simulink model "Citation_FlightGear"  (R2020b)
settings: Solver=ode5  StartTime=0.0  StopTime=100  FixedStep=0.01  RelTol=1e-3  EnableMultiTasking=on
values from neighbouring files (symbols this model uses):
  cv1 = 20000    [gear_params.m]
  cv2 = cv1    (= 20000)    [gear_params.m]
  cv3 = 4000    [gear_params.m]
  cv4 = 20000    [gear_params.m]
  deltagmax1 = 0.25    [gear_params.m]
  deltagmax2 = deltagmax1    (= 0.25)    [gear_params.m]
  deltagmax3 = 0.24    [gear_params.m]
  deltagmax4 = 0.02    [gear_params.m]
  kt1 = 525020    [gear_params.m]
  kt2 = kt1    (= 525020)    [gear_params.m]
  kt3 = 457050    [gear_params.m]
  murol = 0.03*10    (= 0.3)    [gear_params.m]
  P1 = 2000    [gear_params.m]
  P2 = P1    (= 2000)    [gear_params.m]
  P3 = 2550    [gear_params.m]
  P4 = 40000    [gear_params.m]
  xl1 = xcg-6.858    [gear_params.m]
  xl2 = xcg-6.858    [gear_params.m]
  xl3 = xcg-2.0752    [gear_params.m]
  xl4 = xcg-12.742    [gear_params.m]
  yl1 = 1.918    [gear_params.m]
  yl2 = -1.918    [gear_params.m]
  yl3 = 0    [gear_params.m]
  yl4 = 0    [gear_params.m]
  zl1 = zcg-1.701    [gear_params.m]
  zl2 = zcg-1.701    [gear_params.m]
  zl3 = zcg-1.7488    [gear_params.m]
  zl4 = zcg-2.78    [gear_params.m]
undefined symbols (not defined in the file or in its folder): chord, Deng, ealphag, ealphas, Earth, g0, hDME, hGS, lh, massinit, matbuaf, matdaf, matdam, matdbbf, matdeaf, matdgaf, matdqaf, matduaf, matdwaw, matedhr, mateif, matelhr, matemhr, matemv1, matemv2, matemve, matetam, mateuaf, matfaaf, matfaxl, matff, matibaf, matibb, matibmh, matipaf, matipmh, matiraf, matiuaf, matiwaf, matlaf, matlam, matleaf, matleam, matlgaf, matlqaf, matluaf, matmaaf, matmaam, matmaf, matmam, matmbbf, matmeaf, matmeam, matmgaf, matmqaf, matmrbr, matn1d, matn2d, matnbab, matnbaf ... (+55)
libraries: aerolibfltsims x3, aerolibconvert2 x2, aerolibtransform2 x1, aerolibobsolete x1, vrlib x1, aerolibanimutils x1
(part 1 of 5)
settings Model: ExtModeTrigMode=oneshot  ExtModeArmWhenConnect=off  Creator=laurensvaneykeren  LastModifiedBy=ccdevisser
settings DataIOCC: SaveFormat=Array  SignalLoggingSaveFormat=ModelDataLogs  ReturnWorkspaceOutputs=off  SignalLoggingName=sigsOut
settings OptimizationCC: BooleanDataType=off  ExpressionDepthLimit=2147483647  LifeSpan=inf
settings DebuggingCC: SaveWithParameterizedLinksMsg=none  UnderspecifiedInitializationDetection=Classic  MergeDetectMultiDrivingBlocksExec=none  SignalResolutionControl=TryResolveAllWithWarning  MultiTaskDSMMsg=warning  MultiTaskCondExecSysMsg=none  FcnCallInpInsideContextMsg=warning  StateNameClashWarn=warning  SFUnexpectedBacktrackingDiag=warning  SFNoUnconditionalDefaultTransitionDiag=warning  SFExecutionAtInitializationDiag=none  ArithmeticOperatorsInVariantConditions=warning
settings HardwareCC: ProdBitPerPointer=32  ProdBitPerSizeT=32  ProdBitPerPtrDiffT=32  ProdLargestAtomicFloat=None  ProdIntDivRoundTo=Undefined  ProdEndianess=Unspecified  ProdWordSize=32  ProdHWDeviceType=32-bit Generic  TargetUnknown=on
settings ModelReferenceCC: PropagateSignalLabelsOutOfModel=off
settings SFSimCC: SimUseLocalCustomCode=off  CustomCodeUndefinedFunction=UseInterfaceOnly
settings RTWCC: SystemTargetFile=grt_malloc.tlc  GenCodeOnly=on  TemplateMakefile=grt_malloc_default_tmf  RTWUseLocalCustomCode=off
settings CodeAppCC: StateflowObjectComments=on
settings GRTTargetCC: TargetLangStandard=C89/C90 (ANSI)  CombineOutputUpdateFcns=off  GRTInterface=on  UseMalloc=on
settings ConfigComp: CovMetricSettings=dw  CovSaveCumulativeToWorkspaceVar=on  CovSaveSingleToWorkspaceVar=on

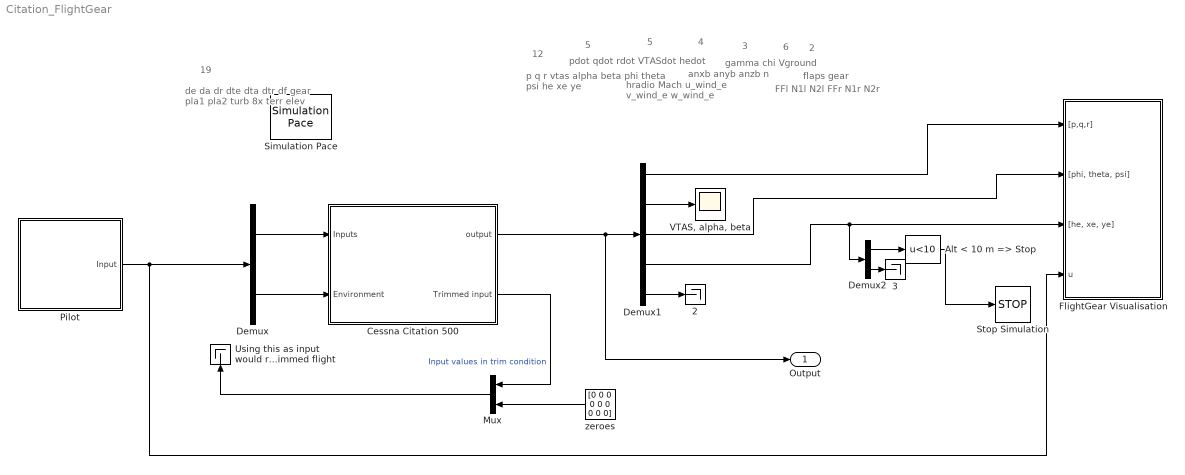
== system Citation_FlightGear ==
  note: de
      | da
      | dr
      | dte
      | dta
      | dtr
      | df
      | gear
      | pla1
      | pla2
      | turb 8x
      | terr elev
  note: p
      | q
      | r
      | vtas
      | alpha
      | beta
      | phi
      | theta
      | psi
      | he
      | xe
      | ye
  note: pdot
      | qdot
      | rdot
      | VTASdot
      | hedot
  note: hradio
      | Mach
      | u_wind_e
      | v_wind_e
      | w_wind_e
  note: anxb
      | anyb
      | anzb
      | n
  note: gamma
      | chi
      | Vground
  note: flaps
      | gear
  note: FFl
      | N1l
      | N2l
      | FFr
      | N1r
      | N2r
  note: 12
  note: 5
  note: 5
  note: 4
  note: 3
  note: 6
  note: 2
  note: 19
  2 : Terminator
  3 : Terminator
  Alt < 10 m => Stop : Fcn  Expr=u<10
  Cessna Citation 500 : Subsystem  mask(Citation Aircraft Model){trimdatafile=CitTrim_V140_H10500_M5300.tri}
      mask prompts: trimdatafile "Trim Condition"
      mask init:
      | initcit;
      mask Display:
      | image(imread('Citation.jpg'))
      | port_label('input', 1, 'Inputs')
      | port_label('input', 2, 'Environment')
      | port_label('output', 1, 'Outputs')
      | port_label('output', 2, 'Trim inputs')
  Demux : Demux  Outputs=[10 9]
      settings: DisplayOption=none
  Demux1 : Demux  Outputs=[3 3 3 3 25]
      settings: DisplayOption=none
  Demux2 : Demux  Outputs=[1 2]
  FlightGear Visualisation : Subsystem
  Mux : Mux  Inputs=2
  Pilot : Subsystem
  Simulation Pace : aerolibanimutils/Simulation Pace  SimulationPace=1  SleepMode=MATLAB Thread  OutputPaceError=off  SampleTime=-1
      settings: AttributesFormatString=%<SimulationPace> sec/sec
  Stop Simulation : Stop
  Using this as input would result in trimmed flight : Terminator
  "VTAS, alpha, beta" : Scope
  zeroes : Constant  Value=[0 0 0 0 0 0 0 0 0]
  Output : Outport
  wires:
  Demux/1 -> Cessna Citation 500/1(Inputs)
  Cessna Citation 500/1(output) -> Demux1/1, Output/1
  Demux/2 -> Cessna Citation 500/2(Environment)
  Cessna Citation 500/2(Trimmed input) -> Mux/1  "Input values in trim condition"
  zeroes/1 -> Mux/2
  Mux/1 -> Using this as input would result in trimmed flight/1
  Demux1/1 -> FlightGear Visualisation/1("[p,q,r]")
  Demux1/2 -> "VTAS, alpha, beta"/1
  Alt < 10 m => Stop/1 -> Stop Simulation/1
  Demux1/5 -> 2/1
  Demux1/4 -> Demux2/1, FlightGear Visualisation/3("[he, xe, ye]")
  Demux2/1 -> Alt < 10 m => Stop/1
  Pilot/1(Input) -> FlightGear Visualisation/4(u), Demux/1
  Demux2/2 -> 3/1
  Demux1/3 -> FlightGear Visualisation/2(" [phi, theta, psi]")

== system Citation_FlightGear/Cessna Citation 500 ==
  note: p
      | q
      | r
      | vtas
      | alpha
      | beta
      | phi
      | theta
      | psi
      | he
      | xe
      | ye
  note: de
      | da
      | dr
      | dte
      | dta
      | dtr
      | df
      | gear
      | pla1
      | pla2
  note: pdot
      | qdot
      | rdot
      | VTASdot
      | hedot
  note: hradio
      | Mach
      | u_wind_e
      | v_wind_e
      | w_wind_e
  note: anxb
      | anyb
      | anzb
      | n
  note: gamma
      | chi
      | Vground
  note: turb 8x
      | terr_elev
  note: flaps
      | gear
  note: de
      | da
      | dr
      | dte
      | dta
      | dtr
      | df
      | gear
      | pla1
      | pla2
  note: FFl
      | N1l
      | N2l
      | FFr
      | N1r
      | N2r
  Inputs : Inport
  Environment : Inport  Port=2
  Actuators : Subsystem
  Citation model DASMAT : Subsystem
  Controllers : Subsystem
  Demux4 : Demux  Outputs=[8 2]
      settings: DisplayOption=none
  Mux1 : Mux  Inputs=7
  Mux2 : Mux  Inputs=2
  trim conditions : Subsystem
  ua sel : Selector  IndexOptions=Index vector (dialog)  Indices=[5 6]  OutputSizes=1
  xdot sel : Selector  IndexOptions=Index vector (dialog)  Indices=[1 2 3 4 10]  OutputSizes=1
  yacc sel : Selector  IndexOptions=Index vector (dialog)  Indices=[4 5 6 15]  OutputSizes=1
  yair sel : Selector  IndexOptions=Index vector (dialog)  Indices=[6 9 22 23 24]  OutputSizes=1
  yfp sel : Selector  IndexOptions=Index vector (dialog)  Indices=[1 2 15]  OutputSizes=1
  ypp sel : Selector  IndexOptions=Index vector (dialog)  Indices=[2 3 4 13 14 15]  OutputSizes=1
  output : Outport
  Trimmed input : Outport  Port=2
  wires:
  Mux1/1 -> output/1
  Citation model DASMAT/1(x) -> Mux1/1, Controllers/1(state)
  Inputs/1 -> Controllers/2(inputs)
  Demux4/1 -> Citation model DASMAT/1(ua), ua sel/1
  Demux4/2 -> Citation model DASMAT/2(ut)
  Environment/1 -> Citation model DASMAT/3(Environment)
  Citation model DASMAT/3(yair) -> yair sel/1
  yair sel/1 -> Mux1/3
  Citation model DASMAT/2(xdot) -> xdot sel/1
  xdot sel/1 -> Mux1/2
  yacc sel/1 -> Mux1/4
  Citation model DASMAT/4(yacc) -> yacc sel/1
  yfp sel/1 -> Mux1/5
  Citation model DASMAT/5(yfp) -> yfp sel/1
  Actuators/1(Out) -> Demux4/1
  trim conditions/1(ua) -> Mux2/1
  trim conditions/2(ut) -> Mux2/2
  Mux2/1 -> Trimmed input/1
  Controllers/1(control inputs) -> Actuators/1(In)
  ua sel/1 -> Mux1/7
  Citation model DASMAT/6(ypp) -> ypp sel/1
  ypp sel/1 -> Mux1/6

== system Citation_FlightGear/FlightGear Visualisation ==
  "[p,q,r]" : Inport
  " [phi, theta, psi]" : Inport  Port=2
  "[he, xe, ye]" : Inport  Port=3
  u : Inport  Port=4
  Constant : Constant  Value=114
  Generate Run Script : aerolibfltsims/Generate Run Script  Architecture=Win64  dataFlow=Send  GeometryModelName=Yak-36  AirportId=KSFO  RunwayId=10L  InitialAltitude=7224  InitialHeading=113  OffsetDistance=4.72  OffsetAzimuth=0  InstallScenery=off  DisableShaders=off  OriginAddress=127.0.0.1  DestinationPort=5502  OriginPort=5505  LocalAddress=127.0.0.1  OutputFileName=runfg30.bat  FlightGearBaseDirectory=D:\Program Files\FlightGear3.0
  "P, Q, R" : Scope
  Send net_fdm Packet to FlightGear : aerolibfltsims/Send net_fdm Packet to FlightGear  DestinationIpAddress=127.0.0.1  DestinationPort=5502  LocalIpPort=-1  varLen=off  SampleTime=-1
      settings: SourceProductBaseCode=AE
  Subsystem : Subsystem
  Sum1 : Sum  Inputs=|++
  phi,theta,psi : Scope
  "posN,posE, h, offsets" : Constant  Value=[0 -1000 12000]
  posN,posE,h : Scope
  wires:
  "posN,posE, h, offsets"/1 -> Sum1/2
  Sum1/1 -> posN,posE,h/1, Subsystem/3(Xe)
  Constant/1 -> Subsystem/4(href)
  u/1 -> Subsystem/5(u)
  Subsystem/1(FG Packet) -> Send net_fdm Packet to FlightGear/1
  "[he, xe, ye]"/1 -> Sum1/1
  "[p,q,r]"/1 -> "P, Q, R"/1, Subsystem/1(pqr)
  " [phi, theta, psi]"/1 -> phi,theta,psi/1, Subsystem/2(phi theta psi)

== system Citation_FlightGear/Pilot ==
  note: Should have 19 elements
  note: de
      | da
      | dr
      | dte
      | dta
      | dtr
      | df
      | gear
      | pla1
      | pla2
      | turb 8x
      | terr elev
  Input Selector Switch : ManualSwitch  CurrentSetting=0
  Joystick : Subsystem
  Mux : Mux  Inputs=12
  Mux1 : Mux  Inputs=12
  Virtual Joystick : Subsystem
  da trim : Constant  Value=0
  da trim1 : Constant  Value=0
  de trim : Constant  Value=0
  de trim1 : Constant  Value=0
  delta flaps : Constant  Value=0
  delta flaps1 : Constant  Value=0
  dr trim : Constant  Value=0
  dr trim1 : Constant  Value=0
  gear (ON=1/OFF=0) : Constant  Value=0
  gear (ON=1/OFF=0)1 : Constant  Value=0
  terr elev : Constant  Value=0
  terr elev1 : Constant  Value=0
  turb 8x : Constant  Value=zeros(1,8)
  turb 8x1 : Constant  Value=zeros(1,8)
  Input : Outport
  wires:
  Joystick/1(delta elevator) -> Mux/1
  Joystick/3(delta rudder) -> Mux/3
  da trim/1 -> Mux/5
  de trim/1 -> Mux/4
  Joystick/2(delta aileron) -> Mux/2
  turb 8x/1 -> Mux/11
  terr elev/1 -> Mux/12
  Joystick/4(Throttle setting) -> Mux/10, Mux/9
  gear (ON=1/OFF=0)/1 -> Mux/8
  dr trim/1 -> Mux/6
  delta flaps/1 -> Mux/7
  Input Selector Switch/1 -> Input/1
  Mux1/1 -> Input Selector Switch/2  "Virtual joystick input"
  dr trim1/1 -> Mux1/6
  gear (ON=1/OFF=0)1/1 -> Mux1/8
  de trim1/1 -> Mux1/4
  delta flaps1/1 -> Mux1/7
  da trim1/1 -> Mux1/5
  turb 8x1/1 -> Mux1/11
  terr elev1/1 -> Mux1/12
  Virtual Joystick/1(Signal 1) -> Mux1/1
  Virtual Joystick/2(Signal 2) -> Mux1/2
  Virtual Joystick/3(Signal 3) -> Mux1/3
  Virtual Joystick/4(Signal 4) -> Mux1/9, Mux1/10
  Mux/1 -> Input Selector Switch/1

== system Citation_FlightGear/Cessna Citation 500/Actuators ==
  note: de
      | da
      | dr
      | dte
      | dta
      | dtr
      | df
      | gear
      | pla1
      | pla2
  note: de
      | da
      | dr
      | dte
      | dta
      | dtr
      | df
      | gear
      | pla1
      | pla2
  In : Inport
  Demux : Demux  Outputs=10
      settings: DisplayOption=none
  Mux : Mux  Inputs=10
  da : Subsystem
  da limits : Saturate  UpperLimit=0.65  LowerLimit=-0.65
  de : Subsystem
  de limits : Saturate  UpperLimit=0.26  LowerLimit=-0.35
  dr : Subsystem
  dr limits : Saturate  UpperLimit=0.38  LowerLimit=-0.38
  flaps : Subsystem
  gear : Subsystem
  Out : Outport
  wires:
  In/1 -> Demux/1
  Mux/1 -> Out/1
  Demux/1 -> de/1(In)
  Demux/2 -> da/1(In)
  Demux/3 -> dr/1(In)
  de/1(Out) -> de limits/1
  da/1(Out) -> da limits/1
  da limits/1 -> Mux/2
  dr/1(Out) -> dr limits/1
  dr limits/1 -> Mux/3
  de limits/1 -> Mux/1
  Demux/8 -> gear/1(In)
  Demux/7 -> flaps/1(In)
  Demux/9 -> Mux/9
  Demux/10 -> Mux/10
  flaps/1(Out) -> Mux/7
  gear/1(Out) -> Mux/8
  Demux/4 -> Mux/4
  Demux/5 -> Mux/5
  Demux/6 -> Mux/6

== system Citation_FlightGear/Cessna Citation 500/Citation model DASMAT ==
  ua : Inport
  ut : Inport  Port=2
  Environment : Inport  Port=3
  AIRCRAFT MODEL : Subsystem
  Mux1 : Mux  Inputs=[8 2 8 12 8]
  Terminator_{16..19} (4 alike) : Terminator
  massinit : Constant  Value=massinit
  x : Outport
  xdot : Outport  Port=2
  yair : Outport  Port=3
  yacc : Outport  Port=4
  yfp : Outport  Port=5
  ypp : Outport  Port=6
  wires:
  AIRCRAFT MODEL/13(FMt) -> Terminator_19/1
  Mux1/1 -> yair/1
  AIRCRAFT MODEL/12(FMag) -> Terminator_17/1
  AIRCRAFT MODEL/11(FMa) -> Terminator_18/1
  AIRCRAFT MODEL/7(gust) -> Mux1/5
  AIRCRAFT MODEL/6(wind) -> Mux1/4
  AIRCRAFT MODEL/5(yad2) -> Mux1/3
  AIRCRAFT MODEL/4(yad1) -> Mux1/2
  AIRCRAFT MODEL/3(yatm) -> Mux1/1
  AIRCRAFT MODEL/2(xdot) -> xdot/1
  AIRCRAFT MODEL/1(x) -> x/1
  AIRCRAFT MODEL/10(ys) -> Terminator_16/1
  AIRCRAFT MODEL/9(yfp) -> yfp/1
  AIRCRAFT MODEL/8(yacc) -> yacc/1
  massinit/1 -> AIRCRAFT MODEL/3(massinit)
  ut/1 -> AIRCRAFT MODEL/2(ut)
  ua/1 -> AIRCRAFT MODEL/1(ua)
  Environment/1 -> AIRCRAFT MODEL/4(Environment)
  AIRCRAFT MODEL/14(ypp) -> ypp/1

== system Citation_FlightGear/Cessna Citation 500/Controllers ==
  state : Inport
  inputs : Inport  Port=2
  A/T disabled : Gain  Gain=0  SaturateOnIntegerOverflow=on  OutDataTypeStr=Inherit: Same as input  ParamDataTypeStr=Inherit: Same as input
  Yaw damper : Subsystem
  add controller outputs to pilot inputs : Sum  Inputs=|+|+|+|  SaturateOnIntegerOverflow=on
  auto throttle : Subsystem
  control inputs : Outport
  wires:
  state/1 -> Yaw damper/1(state), auto throttle/1(state)
  inputs/1 -> Yaw damper/2(inputs), add controller outputs to pilot inputs/3, auto throttle/2(inputs)
  add controller outputs to pilot inputs/1 -> control inputs/1
  Yaw damper/1(controller output) -> add controller outputs to pilot inputs/1
  auto throttle/1(controller output) -> A/T disabled/1
  A/T disabled/1 -> add controller outputs to pilot inputs/2

== system Citation_FlightGear/Cessna Citation 500/trim conditions ==
  PLA1/Tx1 : Constant  Value=ut0(1)
  PLA2/Tx2 : Constant  Value=ut0(2)
  control inputs : Mux  Inputs=8
      settings: DisplayOption=signals
  deltaa : Constant  Value=u0(2)
  deltae : Constant  Value=u0(1)
  deltaf : Constant  Value=u0(7)
  deltar : Constant  Value=u0(3)
  deltata : Constant  Value=u0(5)
  deltate : Constant  Value=u0(4)
  deltatr : Constant  Value=u0(6)
  engine inputs : Mux  Inputs=2
      settings: DisplayOption=signals
  lgsw : Constant  Value=u0(8)
  ua : Outport
  ut : Outport  Port=2
  wires:
  deltaf/1 -> control inputs/7  "df"
  engine inputs/1 -> ut/1
  deltatr/1 -> control inputs/6  "dtr"
  deltata/1 -> control inputs/5  "dta"
  control inputs/1 -> ua/1
  PLA1/Tx1/1 -> engine inputs/1  "pla1"
  PLA2/Tx2/1 -> engine inputs/2  "pla2"
  deltae/1 -> control inputs/1  "de"
  deltaa/1 -> control inputs/2  "da"
  deltar/1 -> control inputs/3  "dr"
  deltate/1 -> control inputs/4  "dte"
  lgsw/1 -> control inputs/8  "lg"

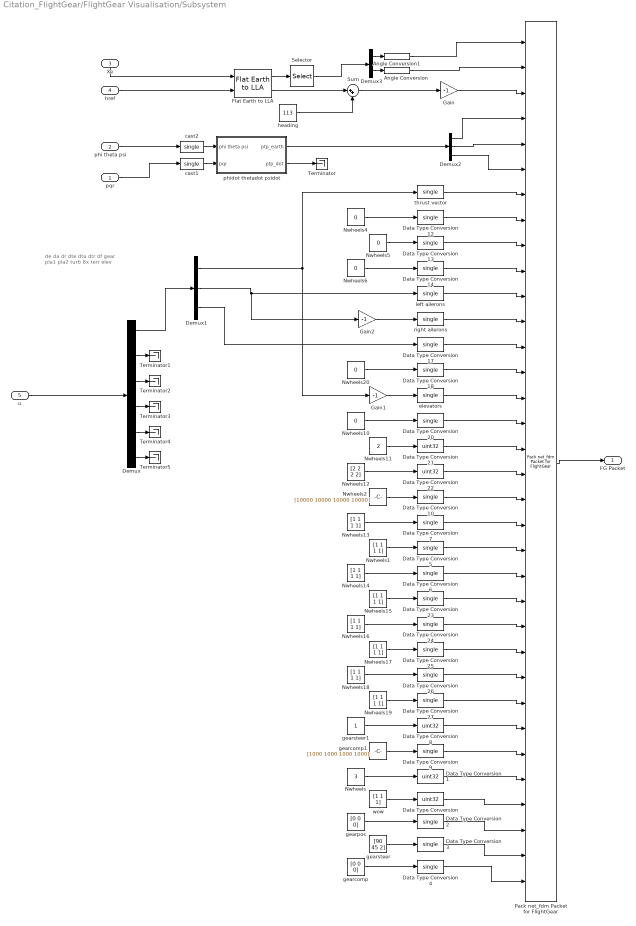
== system Citation_FlightGear/FlightGear Visualisation/Subsystem ==
  note: de
      | da
      | dr
      | dte
      | dta
      | dtr
      | df
      | gear
      | pla1
      | pla2
      | turb 8x
      | terr elev
  pqr : Inport
  phi theta psi : Inport  Port=2
  Xe : Inport  Port=3
  href : Inport  Port=4
  u : Inport  Port=5
  Angle Conversion : aerolibconvert2/Angle Conversion  IU=deg  OU=rad
  Angle Conversion1 : aerolibconvert2/Angle Conversion  IU=deg  OU=rad
  Data Type Conversion{,1,8,21..22} (5 alike) : DataTypeConversion  OutDataTypeStr=uint32
  Data Type Conversion{2..7,9..10,12..14,17..18,20,23..27} (19 alike) : DataTypeConversion  OutDataTypeStr=single
  Demux : Demux  Outputs=[3 3 1 1 2 9]
  Demux1 : Demux  Outputs=[1 1 1]
  Demux2 : Demux  Outputs=3
  Demux3 : Demux  Outputs=2
  Flat Earth to LLA : aerolibtransform2/Flat Earth to LLA  units=Metric (MKS)  ptype=Earth (WGS84)  F=1/298.257223563  R=6378137  refPosPort=off  LL0=[37.7889 -122.4778]  psi=0
  Gain : Gain  Gain=-1
  Gain1 : Gain  Gain=-1
  Gain2 : Gain  Gain=-1
  Nwheels : Constant  Value=3
  Nwheels{1,13..19} (8 alike) : Constant  Value=[1 1 1 1]
  Nwheels{4..6,10,20} (5 alike) : Constant  Value=0
  Nwheels11 : Constant  Value=2
  Nwheels12 : Constant  Value=[2 2 2 2]
  Nwheels2 : Constant  Value=[10000 10000 10000 10000]
  Pack net_fdm Packet for FlightGear : aerolibfltsims/Pack net_fdm Packet for FlightGear  FlightGearVersion=v2016.1  ShowPositionAttitudeInputs=on  ShowVelocityAccelerationInputs=off  ShowControlSurfacePositionInputs=on  ShowEngineFuelInputs=on  ShowLandingGearInputs=on  ShowEnvironmentInputs=off  SampleTime=-1  packetVersion=24
      settings: SourceProductBaseCode=AE
  Selector : Selector  InputPortWidth=2  IndexOptions=Index vector (dialog)  Indices=[2 1]  OutputSizes=1
  Sum : Sum  Inputs=|++
  Terminator{,1..5} (6 alike) : Terminator
  cast1 : DataTypeConversion  OutDataTypeStr=single  SaturateOnIntegerOverflow=on
  cast2 : DataTypeConversion  OutDataTypeStr=single  SaturateOnIntegerOverflow=on
  elevators : DataTypeConversion  OutDataTypeStr=single
  gearcomp : Constant  Value=[0 0 0]
  gearcomp1 : Constant  Value=[1000 1000 1000 1000]
  gearpos : Constant  Value=[0 0 0]  VectorParams1D=off
  gearsteer : Constant  Value=[90 45 2]
  gearsteer1 : Constant
  heading : Constant  Value=113
  left ailerons : DataTypeConversion  OutDataTypeStr=single
  phidot thetadot psidot : Subsystem
  right ailerons : DataTypeConversion  OutDataTypeStr=single
  thrust vector : DataTypeConversion  OutDataTypeStr=single
  wow : Constant  Value=[1 1 1]
  FG Packet : Outport  VectorParamsAs1DForOutWhenUnconnected=off
  wires:
  Pack net_fdm Packet for FlightGear/1 -> FG Packet/1
  href/1 -> Flat Earth to LLA/2
  Flat Earth to LLA/1 -> Selector/1
  Selector/1 -> Demux3/1
  Demux3/1 -> Angle Conversion1/1
  Demux3/2 -> Angle Conversion/1
  Flat Earth to LLA/2 -> Sum/1
  Angle Conversion1/1 -> Pack net_fdm Packet for FlightGear/1
  phidot thetadot psidot/1(ptp_earth) -> Demux2/1
  Demux2/1 -> Pack net_fdm Packet for FlightGear/4
  Demux2/2 -> Pack net_fdm Packet for FlightGear/5
  Demux2/3 -> Pack net_fdm Packet for FlightGear/6
  phidot thetadot psidot/2(ptp_dot) -> Terminator/1
  pqr/1 -> cast1/1
  heading/1 -> Sum/2
  Angle Conversion/1 -> Pack net_fdm Packet for FlightGear/2
  Sum/1 -> Gain/1
  Gain/1 -> Pack net_fdm Packet for FlightGear/3
  Data Type Conversion17/1 -> Pack net_fdm Packet for FlightGear/13
  Data Type Conversion8/1 -> Pack net_fdm Packet for FlightGear/28
  Nwheels13/1 -> Data Type Conversion7/1
  Data Type Conversion25/1 -> Pack net_fdm Packet for FlightGear/25
  left ailerons/1 -> Pack net_fdm Packet for FlightGear/11
  Nwheels15/1 -> Data Type Conversion23/1
  Nwheels19/1 -> Data Type Conversion27/1
  Data Type Conversion12/1 -> Pack net_fdm Packet for FlightGear/8
  Data Type Conversion9/1 -> Pack net_fdm Packet for FlightGear/29
  Demux1/2 -> Gain2/1, left ailerons/1
  Data Type Conversion21/1 -> Pack net_fdm Packet for FlightGear/17
  Data Type Conversion14/1 -> Pack net_fdm Packet for FlightGear/10
  Data Type Conversion6/1 -> Pack net_fdm Packet for FlightGear/22
  thrust vector/1 -> Pack net_fdm Packet for FlightGear/7
  Nwheels6/1 -> Data Type Conversion14/1
  Nwheels12/1 -> Data Type Conversion22/1
  Nwheels14/1 -> Data Type Conversion6/1
  Nwheels5/1 -> Data Type Conversion13/1
  right ailerons/1 -> Pack net_fdm Packet for FlightGear/12
  Data Type Conversion22/1 -> Pack net_fdm Packet for FlightGear/18
  gearcomp1/1 -> Data Type Conversion9/1
  Data Type Conversion13/1 -> Pack net_fdm Packet for FlightGear/9
  Data Type Conversion26/1 -> Pack net_fdm Packet for FlightGear/26
  Nwheels1/1 -> Data Type Conversion5/1
  gearsteer1/1 -> Data Type Conversion8/1
  elevators/1 -> Pack net_fdm Packet for FlightGear/15
  Data Type Conversion18/1 -> Pack net_fdm Packet for FlightGear/14
  Data Type Conversion20/1 -> Pack net_fdm Packet for FlightGear/16
  Nwheels2/1 -> Data Type Conversion10/1
  Nwheels10/1 -> Data Type Conversion20/1
  Xe/1 -> Flat Earth to LLA/1
  Data Type Conversion10/1 -> Pack net_fdm Packet for FlightGear/19
  Nwheels4/1 -> Data Type Conversion12/1
  Data Type Conversion27/1 -> Pack net_fdm Packet for FlightGear/27
  Data Type Conversion4/1 -> Pack net_fdm Packet for FlightGear/34
  gearpos/1 -> Data Type Conversion2/1
  Data Type Conversion2/1 -> Pack net_fdm Packet for FlightGear/32
  Data Type Conversion3/1 -> Pack net_fdm Packet for FlightGear/33
  Nwheels/1 -> Data Type Conversion1/1
  wow/1 -> Data Type Conversion/1
  gearsteer/1 -> Data Type Conversion3/1
  Data Type Conversion1/1 -> Pack net_fdm Packet for FlightGear/30
  gearcomp/1 -> Data Type Conversion4/1
  Data Type Conversion/1 -> Pack net_fdm Packet for FlightGear/31
  Nwheels17/1 -> Data Type Conversion25/1
  Nwheels16/1 -> Data Type Conversion24/1
  Data Type Conversion23/1 -> Pack net_fdm Packet for FlightGear/23
  Data Type Conversion24/1 -> Pack net_fdm Packet for FlightGear/24
  Nwheels11/1 -> Data Type Conversion21/1
  Data Type Conversion7/1 -> Pack net_fdm Packet for FlightGear/20
  Data Type Conversion5/1 -> Pack net_fdm Packet for FlightGear/21
  Nwheels18/1 -> Data Type Conversion26/1
  cast2/1 -> phidot thetadot psidot/1(phi theta psi)
  cast1/1 -> phidot thetadot psidot/2(pqr)
  phi theta psi/1 -> cast2/1
  Demux1/3 -> Data Type Conversion17/1
  Nwheels20/1 -> Data Type Conversion18/1
  u/1 -> Demux/1
  Gain1/1 -> elevators/1
  Demux1/1 -> Gain1/1, thrust vector/1
  Demux/1 -> Demux1/1
  Gain2/1 -> right ailerons/1
  Demux/2 -> Terminator1/1
  Demux/3 -> Terminator2/1
  Demux/4 -> Terminator3/1
  Demux/5 -> Terminator4/1
  Demux/6 -> Terminator5/1

== system Citation_FlightGear/Pilot/Joystick ==
  note: raw inputs
      | aileron [-0.6328,0.014,0.72] right+
      | elevator [-0.6973,-0.033,0.5725] backwards+
      | throttle [-0.6407,0,0.5317]bacwards+
      | rudder [-0.56,0.127,0.73] right+
  note: normalize inputs
      | aileron [-1,0,1] left+
      | elevator [-1,0,1] forward+
      | rudder [-1,0,1] left+
      | throttle [-1,0,1] forward+
  note: apply real limits
      | [deg]
      | [%]
  note: Convert to radians
      | [rad]
      | [%]
  Constant : Constant  Value=0
  Constant1 : Constant  Value=0
  Constant2 : Constant
  Constant3 : Constant  Value=0
  Dead Zone : DeadZone  LowerValue=-0.01  UpperValue=0.01  SaturateOnIntegerOverflow=on
  Dead Zone1 : DeadZone  LowerValue=-0.01  UpperValue=0.01  SaturateOnIntegerOverflow=on
  Dead Zone2 : DeadZone  LowerValue=-0.01  UpperValue=0.01  SaturateOnIntegerOverflow=on
  Demux1 : Demux
      settings: DisplayOption=none
  Gain : Gain  Gain=-1  SaturateOnIntegerOverflow=on  OutDataTypeStr=Inherit: Same as input  ParamDataTypeStr=Inherit: Same as input
  Gain1 : Gain  Gain=-1  SaturateOnIntegerOverflow=on  OutDataTypeStr=Inherit: Same as input  ParamDataTypeStr=Inherit: Same as input
  Gain11 : Gain  Gain=pi/180  SaturateOnIntegerOverflow=on  OutDataTypeStr=Inherit: Same as input  ParamDataTypeStr=Inherit: Same as input
  Gain2 : Gain  Gain=-0.5  SaturateOnIntegerOverflow=on  OutDataTypeStr=Inherit: Same as input  ParamDataTypeStr=Inherit: Same as input
  Gain3 : Gain  Gain=-1  SaturateOnIntegerOverflow=on  OutDataTypeStr=Inherit: Same as input  ParamDataTypeStr=Inherit: Same as input
  Gain4 : Gain  Gain=37.24  SaturateOnIntegerOverflow=on  OutDataTypeStr=Inherit: Same as input  ParamDataTypeStr=Inherit: Same as input
  Gain5 : Gain  Gain=20  SaturateOnIntegerOverflow=on  OutDataTypeStr=Inherit: Same as input  ParamDataTypeStr=Inherit: Same as input
  Gain6 : Gain  SaturateOnIntegerOverflow=on  OutDataTypeStr=Inherit: Same as input  ParamDataTypeStr=Inherit: Same as input
  Gain7 : Gain  Gain=22  SaturateOnIntegerOverflow=on  OutDataTypeStr=Inherit: Same as input  ParamDataTypeStr=Inherit: Same as input
  Gain8 : Gain  Gain=pi/180  SaturateOnIntegerOverflow=on  OutDataTypeStr=Inherit: Same as input  ParamDataTypeStr=Inherit: Same as input
  Gain9 : Gain  Gain=pi/180  SaturateOnIntegerOverflow=on  OutDataTypeStr=Inherit: Same as input  ParamDataTypeStr=Inherit: Same as input
  Joystick Input : vrlib/Joystick Input  joyid=1  adjustports=on  forcefeed=off
  Scope{,1..3} (4 alike) : Scope
  Sum{,1..3} (4 alike) : Sum  Inputs=-+|  SaturateOnIntegerOverflow=on
  Terminator3 : Terminator
  delta elevator : Outport
  delta aileron : Outport  Port=2
  delta rudder : Outport  Port=3
  Throttle setting : Outport  Port=4
  wires:
  Joystick Input/1 -> Demux1/1
  Joystick Input/2 -> Terminator3/1
  Demux1/1 -> Sum/2
  Constant/1 -> Sum/1
  Constant1/1 -> Sum1/1
  Demux1/2 -> Sum1/2
  Constant2/1 -> Sum2/1
  Constant3/1 -> Sum3/1
  Sum/1 -> Dead Zone/1
  Gain/1 -> Gain4/1
  Sum1/1 -> Dead Zone1/1
  Gain1/1 -> Gain5/1
  Sum2/1 -> Gain2/1
  Sum3/1 -> Dead Zone2/1
  Gain3/1 -> Gain7/1
  Gain4/1 -> Gain8/1
  Gain5/1 -> Gain9/1
  Gain6/1 -> Scope2/1, Throttle setting/1
  Gain7/1 -> Gain11/1
  Gain8/1 -> Scope/1, delta aileron/1
  Gain9/1 -> Scope1/1, delta elevator/1
  Gain11/1 -> Scope3/1, delta rudder/1
  Gain2/1 -> Gain6/1
  Demux1/4 -> Sum2/2
  Demux1/3 -> Sum3/2
  Dead Zone/1 -> Gain/1
  Dead Zone1/1 -> Gain1/1
  Dead Zone2/1 -> Gain3/1

== system Citation_FlightGear/Pilot/Virtual Joystick ==
  Throttle setting : Subsystem  Tag=STV Subsys  LoadFcn=sigbuilder_block('load');  StartFcn=sigbuilder_block('start');  StopFcn=sigbuilder_block('stop');  ClipboardFcn=sigbuilder_block('clipboard');  mask(Sigbuilder block){tuvar=[0:10]}
      mask help: Simulink:masks:SigbuilderBlock_MD
      mask init:
      | if ~strcmp(get_param(bdroot(gcbh),'SimulationStatus'),'stopped') tuvar = sigbuilder_block('maskInit'); end
      settings: CopyFcn=sigbuilder_block('copy');  DeleteFcn=sigbuilder_block('delete');  ModelCloseFcn=sigbuilder_block('modelClose');  PreSaveFcn=sigbuilder_block('preSave');  PauseFcn=sigbuilder_block('pause');  ContinueFcn=sigbuilder_block('continue');  NameChangeFcn=sigbuilder_block('namechange');  OpenFcn=sigbuilder_block('open',[437.6 199.2 550.4 400 ]);  CloseFcn=sigbuilder_block('close');
      mask Display: plot(0, 0, 100, 100,[2, 2, 32, 32, 2], [68, 8, 8, 68, 68],[32, 2], [38, 38], [32, 19, 2],[53, 60, 44], [32, 17, 17, 2],[16, 16, 31, 31]);txt = getActiveGroup(gcbh);text(2, 100, txt,'verticalAlignment', 'top');
  delta aileron : Subsystem  Tag=STV Subsys  LoadFcn=sigbuilder_block('load');  StartFcn=sigbuilder_block('start');  StopFcn=sigbuilder_block('stop');  ClipboardFcn=sigbuilder_block('clipboard');  mask(Sigbuilder block){tuvar=[0:10]}
      mask help: Simulink:masks:SigbuilderBlock_MD
      mask init:
      | if ~strcmp(get_param(bdroot(gcbh),'SimulationStatus'),'stopped') tuvar = sigbuilder_block('maskInit'); end
      settings: CopyFcn=sigbuilder_block('copy');  DeleteFcn=sigbuilder_block('delete');  ModelCloseFcn=sigbuilder_block('modelClose');  PreSaveFcn=sigbuilder_block('preSave');  PauseFcn=sigbuilder_block('pause');  ContinueFcn=sigbuilder_block('continue');  NameChangeFcn=sigbuilder_block('namechange');  OpenFcn=sigbuilder_block('open',[437.6 199.2 550.4 400 ]);  CloseFcn=sigbuilder_block('close');
      mask Display: plot(0, 0, 100, 100,[2, 2, 32, 32, 2], [68, 8, 8, 68, 68],[32, 2], [38, 38], [32, 19, 2],[53, 60, 44], [32, 17, 17, 2],[16, 16, 31, 31]);txt = getActiveGroup(gcbh);text(2, 100, txt,'verticalAlignment', 'top');
  delta elevator : Subsystem  Tag=STV Subsys  LoadFcn=sigbuilder_block('load');  StartFcn=sigbuilder_block('start');  StopFcn=sigbuilder_block('stop');  ClipboardFcn=sigbuilder_block('clipboard');  mask(Sigbuilder block){tuvar=[0:10]}
      mask help: Simulink:masks:SigbuilderBlock_MD
      mask init:
      | if ~strcmp(get_param(bdroot(gcbh),'SimulationStatus'),'stopped') tuvar = sigbuilder_block('maskInit'); end
      settings: CopyFcn=sigbuilder_block('copy');  DeleteFcn=sigbuilder_block('delete');  ModelCloseFcn=sigbuilder_block('modelClose');  PreSaveFcn=sigbuilder_block('preSave');  PauseFcn=sigbuilder_block('pause');  ContinueFcn=sigbuilder_block('continue');  NameChangeFcn=sigbuilder_block('namechange');  OpenFcn=sigbuilder_block('open',[437.6 199.2 550.4 400 ]);  CloseFcn=sigbuilder_block('close');
      mask Display: plot(0, 0, 100, 100,[2, 2, 32, 32, 2], [68, 8, 8, 68, 68],[32, 2], [38, 38], [32, 19, 2],[53, 60, 44], [32, 17, 17, 2],[16, 16, 31, 31]);txt = getActiveGroup(gcbh);text(2, 100, txt,'verticalAlignment', 'top');
  delta rudder : Subsystem  Tag=STV Subsys  LoadFcn=sigbuilder_block('load');  StartFcn=sigbuilder_block('start');  StopFcn=sigbuilder_block('stop');  ClipboardFcn=sigbuilder_block('clipboard');  mask(Sigbuilder block){tuvar=[0:10]}
      mask help: Simulink:masks:SigbuilderBlock_MD
      mask init:
      | if ~strcmp(get_param(bdroot(gcbh),'SimulationStatus'),'stopped') tuvar = sigbuilder_block('maskInit'); end
      settings: CopyFcn=sigbuilder_block('copy');  DeleteFcn=sigbuilder_block('delete');  ModelCloseFcn=sigbuilder_block('modelClose');  PreSaveFcn=sigbuilder_block('preSave');  PauseFcn=sigbuilder_block('pause');  ContinueFcn=sigbuilder_block('continue');  NameChangeFcn=sigbuilder_block('namechange');  OpenFcn=sigbuilder_block('open',[437.6 199.2 550.4 400 ]);  CloseFcn=sigbuilder_block('close');
      mask Display: plot(0, 0, 100, 100,[2, 2, 32, 32, 2], [68, 8, 8, 68, 68],[32, 2], [38, 38], [32, 19, 2],[53, 60, 44], [32, 17, 17, 2],[16, 16, 31, 31]);txt = getActiveGroup(gcbh);text(2, 100, txt,'verticalAlignment', 'top');
  Signal 1 : Outport
  Signal 2 : Outport  Port=2
  Signal 3 : Outport  Port=3
  Signal 4 : Outport  Port=4
  wires:
  delta elevator/1(Signal 1) -> Signal 1/1
  delta rudder/1(Signal 1) -> Signal 3/1
  Throttle setting/1(Signal 1) -> Signal 4/1
  delta aileron/1(Signal 1) -> Signal 2/1

== system Citation_FlightGear/Cessna Citation 500/Actuators/da ==
  In : Inport
  Gain : Gain  Gain=13  SaturateOnIntegerOverflow=on  OutDataTypeStr=Inherit: Same as input  ParamDataTypeStr=Inherit: Same as input
  Integrator : Integrator  InitialCondition=u0(2)
  Sum : Sum  Inputs=|+-  SaturateOnIntegerOverflow=on
  Out : Outport
  wires:
  Integrator/1 -> Out/1, Sum/2
  In/1 -> Sum/1
  Sum/1 -> Gain/1
  Gain/1 -> Integrator/1

== system Citation_FlightGear/Cessna Citation 500/Actuators/de ==
  In : Inport
  Gain : Gain  Gain=13  SaturateOnIntegerOverflow=on  OutDataTypeStr=Inherit: Same as input  ParamDataTypeStr=Inherit: Same as input
  Integrator : Integrator  InitialCondition=u0(1)
  Sum : Sum  Inputs=|+-  SaturateOnIntegerOverflow=on
  Out : Outport
  wires:
  Integrator/1 -> Out/1, Sum/2
  In/1 -> Sum/1
  Sum/1 -> Gain/1
  Gain/1 -> Integrator/1

== system Citation_FlightGear/Cessna Citation 500/Actuators/dr ==
  In : Inport
  Gain : Gain  Gain=13  SaturateOnIntegerOverflow=on  OutDataTypeStr=Inherit: Same as input  ParamDataTypeStr=Inherit: Same as input
  Integrator : Integrator  InitialCondition=u0(3)
  Sum : Sum  Inputs=|+-  SaturateOnIntegerOverflow=on
  Out : Outport
  wires:
  Integrator/1 -> Out/1, Sum/2
  In/1 -> Sum/1
  Sum/1 -> Gain/1
  Gain/1 -> Integrator/1

== system Citation_FlightGear/Cessna Citation 500/Actuators/flaps ==
  In : Inport
  Gain : Gain  Gain=0.9  SaturateOnIntegerOverflow=on  OutDataTypeStr=Inherit: Same as input  ParamDataTypeStr=Inherit: Same as input
  Integrator : Integrator  InitialCondition=u0(7)
  Sum : Sum  Inputs=|+-  SaturateOnIntegerOverflow=on
  Out : Outport
  wires:
  Integrator/1 -> Out/1, Sum/2
  In/1 -> Sum/1
  Sum/1 -> Gain/1
  Gain/1 -> Integrator/1

== system Citation_FlightGear/Cessna Citation 500/Actuators/gear ==
  In : Inport
  Gain : Gain  Gain=0.6  SaturateOnIntegerOverflow=on  OutDataTypeStr=Inherit: Same as input  ParamDataTypeStr=Inherit: Same as input
  Integrator : Integrator  InitialCondition=u0(8)
  Sum : Sum  Inputs=|+-  SaturateOnIntegerOverflow=on
  Out : Outport
  wires:
  Integrator/1 -> Out/1, Sum/2
  In/1 -> Sum/1
  Sum/1 -> Gain/1
  Gain/1 -> Integrator/1

== system Citation_FlightGear/Cessna Citation 500/Citation model DASMAT/AIRCRAFT MODEL ==
  ua : Inport
  ut : Inport  Port=2
  massinit : Inport  Port=3
  Environment : Inport  Port=4
  AFM : Subsystem
  AIRDATA : Subsystem
  Demux : Demux  Outputs=[8 1]
      settings: DisplayOption=none
  EFM : Subsystem
  EQM : Subsystem
  FM SORT : Subsystem
  GRAVITY : Subsystem
  LANDING GEAR : Subsystem
  OBSERVATIONS : Subsystem
  WIND/TURBULENCE : Subsystem
  x : Outport
  xdot : Outport  Port=2
  yatm : Outport  Port=3
  yad1 : Outport  Port=4
  yad2 : Outport  Port=5
  wind : Outport  Port=6
  gust : Outport  Port=7
  yacc : Outport  Port=8
  yfp : Outport  Port=9
  ys : Outport  Port=10
  FMa : Outport  Port=11
  FMag : Outport  Port=12
  FMt : Outport  Port=13
  ypp : Outport  Port=14
  wires:
  AFM/1(FMa) -> FM SORT/1(FMa), EQM/2(FMa)
  OBSERVATIONS/3(ys) -> ys/1
  OBSERVATIONS/2(yfp) -> yfp/1
  EQM/4(FMtot corrected) -> OBSERVATIONS/4(FMtot)
  EQM/3(yuvw) -> OBSERVATIONS/3(yuvw)
  EFM/1(FMt) -> FM SORT/3(FMt), FMt/1
  AFM/4(FMag) -> FM SORT/2(FMag), FMag/1
  ua/1 -> AFM/2(ua), LANDING GEAR/4(ua)
  ut/1 -> EFM/2(ut)
  OBSERVATIONS/1(yacc) -> yacc/1
  FM SORT/1(FMtot) -> EQM/1("FMtot ")
  EQM/5(FMa corrected) -> OBSERVATIONS/5(FMa), FMa/1
  AFM/2(FMadot) -> EQM/3(FMadot)
  AFM/3(FMbdot) -> EQM/4(FMbdot)
  GRAVITY/1(Fgr) -> FM SORT/4("Fgr "), OBSERVATIONS/6(Fgr)
  massinit/1 -> EFM/3(massinit), AFM/3(massinit), GRAVITY/2(massinit), EQM/5(massinit), OBSERVATIONS/7(massinit), LANDING GEAR/3(massinit)
  AIRDATA/3(yad2) -> EFM/6(yad2), AFM/5(yad2), yad2/1
  AIRDATA/2(yad1) -> AFM/4(yad1), EFM/5(yad1), yad1/1
  AIRDATA/1(yatm) -> yatm/1, GRAVITY/3(yatm), OBSERVATIONS/8(yatm), EFM/4(yatm), AFM/7(yatm)
  EQM/1(x) -> OBSERVATIONS/1(x), AIRDATA/1(x), WIND/TURBULENCE/1("x "), AFM/1(x), EFM/1(x), GRAVITY/1("x "), LANDING GEAR/1(x), x/1
  WIND/TURBULENCE/1(wind) -> EQM/6(wind), wind/1
  EQM/2(xdot) -> xdot/1, OBSERVATIONS/2(xdot), LANDING GEAR/2(xdot)
  Environment/1 -> Demux/1
  Demux/1 -> gust/1, AFM/6(gust)
  Demux/2 -> AIRDATA/2(terrain elevation), LANDING GEAR/5(terr elev)  "terrain elevation"
  LANDING GEAR/1(Fmt) -> FM SORT/5(Fgear)
  EFM/2(ypp) -> ypp/1

== system Citation_FlightGear/Cessna Citation 500/Controllers/Yaw damper ==
  state : Inport
  inputs : Inport  Port=2
  Gain : Gain  SaturateOnIntegerOverflow=on  OutDataTypeStr=Inherit: Same as input  ParamDataTypeStr=Inherit: Same as input
  Washout : TransferFcn  Numerator=[1 0]  Denominator=[1 1/4]
  dr : Gain  Gain=[0 0 1 0 0 0 0 0 0 0]  SaturateOnIntegerOverflow=on  OutDataTypeStr=Inherit: Same as input  ParamDataTypeStr=Inherit: Same as input
  not used : Terminator
  r  sel : Selector  IndexOptions=Index vector (dialog)  Indices=[3]  OutputSizes=1
  controller output : Outport
  wires:
  Washout/1 -> Gain/1
  dr/1 -> controller output/1
  state/1 -> r  sel/1
  r  sel/1 -> Washout/1  "r"
  inputs/1 -> not used/1
  Gain/1 -> dr/1

== system Citation_FlightGear/Cessna Citation 500/Controllers/auto throttle ==
  state : Inport
  inputs : Inport  Port=2
  Gain : Gain  Gain=0.5  SaturateOnIntegerOverflow=on  OutDataTypeStr=Inherit: Same as input  ParamDataTypeStr=Inherit: Same as input
  Saturation : Saturate  UpperLimit=1.0  LowerLimit=0.0
  Sum : Sum  Inputs=+-|  SaturateOnIntegerOverflow=on
  VTAS ref (trim value) : Constant  Value=x0(4)
  VTAS sel : Selector  IndexOptions=Index vector (dialog)  Indices=[4]  OutputSizes=1
  controller output is later added to pilot input! : Sum  Inputs=|+-  SaturateOnIntegerOverflow=on
  pla1&2 : Gain  Gain=[0 0 0 0 0 0 0 0 1 1]  SaturateOnIntegerOverflow=on  OutDataTypeStr=Inherit: Same as input  ParamDataTypeStr=Inherit: Same as input
  pla1&2 as well : Gain  Gain=[0 0 0 0 0 0 0 0 1 1]  SaturateOnIntegerOverflow=on  OutDataTypeStr=Inherit: Same as input  ParamDataTypeStr=Inherit: Same as input
  controller output : Outport
  wires:
  inputs/1 -> pla1&2 as well/1
  state/1 -> VTAS sel/1
  VTAS sel/1 -> Sum/2  "VTAS"
  VTAS ref (trim value)/1 -> Sum/1
  Sum/1 -> Gain/1
  pla1&2/1 -> controller output is later added to pilot input!/1
  Gain/1 -> Saturation/1
  controller output is later added to pilot input!/1 -> controller output/1
  Saturation/1 -> pla1&2/1
  pla1&2 as well/1 -> controller output is later added to pilot input!/2

== system Citation_FlightGear/FlightGear Visualisation/Subsystem/phidot thetadot psidot ==
  phi theta psi : Inport
  pqr : Inport  Port=2
  Concatenate1 : Concatenate  NumInputs=3
  Concatenate2 : Concatenate  NumInputs=3
  SinCos : aerolibobsolete/SinCos
      settings: SourceProductBaseCode=AE
  phidot : Fcn  Expr=u[1]+(u[2]*u[4]+u[3]*u[7])*(u[5]/u[8])
  psidot : Fcn  Expr=(u[2]*u[4]+u[3]*u[7])/u[8]
  thetadot : Fcn  Expr=u[2]*u[7]-u[3]*u[4]
  ptp_earth : Outport  VectorParamsAs1DForOutWhenUnconnected=off
  ptp_dot : Outport  Port=2  VectorParamsAs1DForOutWhenUnconnected=off
  wires:
  Concatenate1/1 -> psidot/1, phidot/1, thetadot/1
  pqr/1 -> Concatenate1/1
  phi theta psi/1 -> SinCos/1, ptp_earth/1
  psidot/1 -> Concatenate2/3
  thetadot/1 -> Concatenate2/2
  phidot/1 -> Concatenate2/1
  Concatenate2/1 -> ptp_dot/1
  SinCos/1 -> Concatenate1/2
  SinCos/2 -> Concatenate1/3

== system Citation_FlightGear/Pilot/Virtual Joystick/Throttle setting ==
  Demux : Demux  Tag=STV Demux  Outputs=1
      settings: DisplayOption=none
  FromWs : FromWorkspace  Tag=STV FromWs  VariableName=tuvar
      SigBuilderData=|
      | common.afterFinalStr = 'Extrapolate'
      | common.sampleTime = 0
      | dataSet.timeRange = [0 10]
      | dataSet.name = 'Group 1'
      | sbobj.Groups.Name = 'Group 1'
      | sbobj.Groups.Signals.Name = 'Signal 1'
      | sbobj.Groups.Signals.XData = [0 4 4 6 6 10]
      | sbobj.Groups.Signals.YData = [0 0 1 1 0 0]
  Signal 1 : Outport  Tag=STV Outport
  wires:
  Demux/1 -> Signal 1/1
  FromWs/1 -> Demux/1

== system Citation_FlightGear/Pilot/Virtual Joystick/delta aileron ==
  Demux : Demux  Tag=STV Demux  Outputs=1
      settings: DisplayOption=none
  FromWs : FromWorkspace  Tag=STV FromWs  VariableName=tuvar
      SigBuilderData=|
      | common.afterFinalStr = 'Extrapolate'
      | common.sampleTime = 0
      | dataSet.timeRange = [0 10]
      | dataSet.name = 'Group 1'
      | sbobj.Groups.Name = 'Group 1'
      | sbobj.Groups.Signals.Name = 'Signal 1'
      | sbobj.Groups.Signals.XData = [0 4 4 6 6 10]
      | sbobj.Groups.Signals.YData = [0 0 1 1 0 0]
  Signal 1 : Outport  Tag=STV Outport
  wires:
  Demux/1 -> Signal 1/1
  FromWs/1 -> Demux/1

== system Citation_FlightGear/Pilot/Virtual Joystick/delta elevator ==
  Demux : Demux  Tag=STV Demux  Outputs=1
      settings: DisplayOption=none
  FromWs : FromWorkspace  Tag=STV FromWs  VariableName=tuvar
      SigBuilderData=|
      | common.afterFinalStr = 'Extrapolate'
      | common.sampleTime = 0
      | dataSet.timeRange = [0 10]
      | dataSet.name = 'Group 1'
      | sbobj.Groups.Name = 'Group 1'
      | sbobj.Groups.Signals.Name = 'Signal 1'
      | sbobj.Groups.Signals.XData = [0 4 4 6 6 10]
      | sbobj.Groups.Signals.YData = [0 0 1 1 0 0]
  Signal 1 : Outport  Tag=STV Outport
  wires:
  Demux/1 -> Signal 1/1
  FromWs/1 -> Demux/1

== system Citation_FlightGear/Pilot/Virtual Joystick/delta rudder ==
  Demux : Demux  Tag=STV Demux  Outputs=1
      settings: DisplayOption=none
  FromWs : FromWorkspace  Tag=STV FromWs  VariableName=tuvar
      SigBuilderData=|
      | common.afterFinalStr = 'Extrapolate'
      | common.sampleTime = 0
      | dataSet.timeRange = [0 10]
      | dataSet.name = 'Group 1'
      | sbobj.Groups.Name = 'Group 1'
      | sbobj.Groups.Signals.Name = 'Signal 1'
      | sbobj.Groups.Signals.XData = [0 4 4 6 6 10]
      | sbobj.Groups.Signals.YData = [0 0 1 1 0 0]
  Signal 1 : Outport  Tag=STV Outport
  wires:
  Demux/1 -> Signal 1/1
  FromWs/1 -> Demux/1

== system Citation_FlightGear/Cessna Citation 500/Citation model DASMAT/AIRCRAFT MODEL/AFM ==
  x : Inport
  ua : Inport  Port=2
  massinit : Inport  Port=3
  yad1 : Inport  Port=4
  yad2 : Inport  Port=5
  gust : Inport  Port=6
  yatm : Inport  Port=7
  Aero axes-cg transformation : Subsystem
  Aeromod : Subsystem
  FMaerodims : Subsystem
  FMgustdims : Subsystem
  Gust axes-cg transformation : Subsystem
  FMa : Outport
  FMadot : Outport  Port=2
  FMbdot : Outport  Port=3
  FMag : Outport  Port=4
  wires:
  FMaerodims/3(FMbdot) -> FMbdot/1
  FMgustdims/1(FMag) -> FMag/1
  FMaerodims/2(FMadot) -> FMadot/1
  FMaerodims/1(FMa) -> FMa/1
  ua/1 -> Aeromod/2(ua)
  yad2/1 -> Aeromod/5(yad2)
  gust/1 -> Aeromod/6(gust)
  Aero axes-cg transformation/1(Ca) -> FMaerodims/1(Ca)
  Aero axes-cg transformation/2(Cadot) -> FMaerodims/2(Cadot)
  Aero axes-cg transformation/3(Cbdot) -> FMaerodims/3(Cbdot)
  Gust axes-cg transformation/1(Cag) -> FMgustdims/1(Cag)
  yad1/1 -> FMaerodims/5(yad1), FMgustdims/2(yad1), Aeromod/4(yad1)
  massinit/1 -> Aero axes-cg transformation/5(massinit), Gust axes-cg transformation/3(massinit), Aeromod/3(massinit)
  Aeromod/1(Ca) -> Aero axes-cg transformation/1(Ca model)
  Aeromod/2(Cadot) -> Aero axes-cg transformation/2(Cadot model)
  Aeromod/3(Cbdot) -> Aero axes-cg transformation/3(Cbdot model)
  Aeromod/4(Cag) -> Gust axes-cg transformation/1(Cag model)
  x/1 -> Aero axes-cg transformation/4("x "), Gust axes-cg transformation/2("x "), FMaerodims/4(x), Aeromod/1(x)
  yatm/1 -> Aeromod/7(yatm)

== system Citation_FlightGear/Cessna Citation 500/Citation model DASMAT/AIRCRAFT MODEL/AIRDATA ==
  x : Inport
  terrain elevation : Inport  Port=2
  Demux : Demux  Outputs=[8 2 8]
      settings: DisplayOption=none
  Demux1 : Demux  Outputs=[5 1 2]
      settings: DisplayOption=none
  Mux : Mux  Inputs=[5 1 2]
  Sum : Sum  Inputs=-+|  SaturateOnIntegerOverflow=on
  airdata : S-Function  FunctionName=ac_atmos  SFunctionDeploymentMode=off  EnableBusSupport=off
  yatm : Outport
  yad1 : Outport  Port=2
  yad2 : Outport  Port=3
  wires:
  x/1 -> airdata/1
  airdata/1 -> Demux/1
  Demux/2 -> yad1/1
  Demux/3 -> yad2/1
  Demux/1 -> Demux1/1
  Mux/1 -> yatm/1
  Demux1/1 -> Mux/1
  Demux1/3 -> Mux/3
  Demux1/2 -> Sum/2
  Sum/1 -> Mux/2
  terrain elevation/1 -> Sum/1

== system Citation_FlightGear/Cessna Citation 500/Citation model DASMAT/AIRCRAFT MODEL/EFM ==
  x : Inport
  ut : Inport  Port=2
  massinit : Inport  Port=3
  yatm : Inport  Port=4
  yad1 : Inport  Port=5
  yad2 : Inport  Port=6
  Engine axes-cg transformation : Subsystem
  Engmod : Subsystem
  FMt : Outport
  ypp : Outport  Port=2
  wires:
  massinit/1 -> Engine axes-cg transformation/3(massinit)
  Engine axes-cg transformation/1(FMt) -> FMt/1
  ut/1 -> Engmod/2(ut)
  yatm/1 -> Engmod/3(yatm)
  yad2/1 -> Engmod/5(yad2)
  x/1 -> Engine axes-cg transformation/2("x "), Engmod/1(x)
  yad1/1 -> Engmod/4(yad1)
  Engmod/1(FMt) -> Engine axes-cg transformation/1(FMt model)
  Engmod/2(ypp) -> ypp/1

== system Citation_FlightGear/Cessna Citation 500/Citation model DASMAT/AIRCRAFT MODEL/EQM ==
  "FMtot " : Inport
  FMa : Inport  Port=2
  FMadot : Inport  Port=3
  FMbdot : Inport  Port=4
  massinit : Inport  Port=5
  wind : Inport  Port=6
  CFMa correction : Subsystem
  Integrator : Integrator  InitialCondition=x0
  State Derivatives : Subsystem
  x : Outport
  xdot : Outport  Port=2
  yuvw : Outport  Port=3
  FMtot corrected : Outport  Port=4
  FMa corrected : Outport  Port=5
  wires:
  State Derivatives/2(yuvw) -> yuvw/1
  State Derivatives/3(FMtot corrected) -> FMtot corrected/1
  FMa/1 -> CFMa correction/2(FMa)
  State Derivatives/1(xdot) -> xdot/1, CFMa correction/1(xdot), Integrator/1
  CFMa correction/1(FMa corrected) -> FMa corrected/1
  massinit/1 -> State Derivatives/5(massinit)
  "FMtot "/1 -> State Derivatives/2(FMtot)
  FMadot/1 -> CFMa correction/3(FMadot), State Derivatives/3(FMadot)
  FMbdot/1 -> CFMa correction/4(FMbdot), State Derivatives/4(FMbdot)
  Integrator/1 -> State Derivatives/1(x), x/1
  wind/1 -> State Derivatives/6(wind)

== system Citation_FlightGear/Cessna Citation 500/Citation model DASMAT/AIRCRAFT MODEL/FM SORT ==
  FMa : Inport
  FMag : Inport  Port=2
  FMt : Inport  Port=3
  "Fgr " : Inport  Port=4
  Fgear : Inport  Port=5
  Mux : Mux  Inputs=[12 12]
  Sum : Sum  Inputs=+++++  InputSameDT=on  SaturateOnIntegerOverflow=on  OutDataTypeStr=Inherit: Same as first input
  Sum1 : Sum  Inputs=++++  InputSameDT=on  SaturateOnIntegerOverflow=on  OutDataTypeStr=Inherit: Same as first input
  aero : Demux  Outputs=[12 12]
      settings: DisplayOption=none
  engine : Demux  Outputs=[12 12]
      settings: DisplayOption=none
  gear : Demux  Outputs=[12 12]
      settings: DisplayOption=none
  gust : Demux  Outputs=[12 12]
      settings: DisplayOption=none
  FMtot : Outport
  wires:
  FMt/1 -> engine/1
  FMa/1 -> aero/1
  FMag/1 -> gust/1
  gust/2 -> Sum1/2
  Sum1/1 -> Mux/2
  engine/2 -> Sum1/3
  aero/2 -> Sum1/1
  gust/1 -> Sum/2
  engine/1 -> Sum/3
  Sum/1 -> Mux/1
  "Fgr "/1 -> Sum/4
  aero/1 -> Sum/1
  Mux/1 -> FMtot/1
  Fgear/1 -> gear/1
  gear/1 -> Sum/5
  gear/2 -> Sum1/4

== system Citation_FlightGear/Cessna Citation 500/Citation model DASMAT/AIRCRAFT MODEL/GRAVITY ==
  "x " : Inport
  massinit : Inport  Port=2
  yatm : Inport  Port=3
  Fgr transformation : S-Function  FunctionName=ac_axes  Parameters=3  SFunctionDeploymentMode=off  EnableBusSupport=off
  Mux : Mux  Inputs=[12 3]
  Mux1 : Mux  Inputs=3
  Terminator_{1..9} (9 alike) : Terminator
  W : Product  InputSameDT=on  SaturateOnIntegerOverflow=on  OutDataTypeStr=Inherit: Same as first input
  atmosphere : Demux  Outputs=8
      settings: DisplayOption=none
  mass cg inertia : Demux  Outputs=[1 3 4]
      settings: DisplayOption=none
  zero : Constant  Value=0
  Fgr : Outport
  wires:
  mass cg inertia/3 -> Terminator_9/1
  mass cg inertia/2 -> Terminator_8/1
  atmosphere/8 -> Terminator_7/1
  atmosphere/7 -> Terminator_6/1
  atmosphere/6 -> Terminator_5/1
  atmosphere/5 -> Terminator_4/1
  atmosphere/3 -> Terminator_3/1
  atmosphere/2 -> Terminator_2/1
  atmosphere/1 -> Terminator_1/1
  Mux/1 -> Fgr transformation/1
  "x "/1 -> Mux/1
  Fgr transformation/1 -> Fgr/1
  mass cg inertia/1 -> W/1
  massinit/1 -> mass cg inertia/1
  yatm/1 -> atmosphere/1
  W/1 -> Mux1/3
  Mux1/1 -> Mux/2
  zero/1 -> Mux1/1, Mux1/2
  atmosphere/4 -> W/2

== system Citation_FlightGear/Cessna Citation 500/Citation model DASMAT/AIRCRAFT MODEL/LANDING GEAR ==
  note: Landing Gear Model
      | Cessna Citation 500
      | Version 0.04NLR
      | (c) A.R. Veldhuijzen September 2001
  x : Inport
  xdot : Inport  Port=2
  massinit : Inport  Port=3
  ua : Inport  Port=4
  terr elev : Inport  Port=5
  Gear axes-cg transformation : Subsystem
  Landing Gear model : Subsystem
  Switch : Switch  Threshold=0.95  SaturateOnIntegerOverflow=on
  gear position : Selector  IndexOptions=Index vector (dialog)  Indices=[8]  OutputSizes=1
  zero : Constant  Value=[0 0 0 0 0 0]
  Fmt : Outport
  wires:
  xdot/1 -> Landing Gear model/2(xdot)
  x/1 -> Landing Gear model/1(x), Gear axes-cg transformation/2("x ")
  massinit/1 -> Gear axes-cg transformation/3(massinit)
  Gear axes-cg transformation/1(FMt) -> Fmt/1
  zero/1 -> Switch/1
  Landing Gear model/1(Forces and Moments) -> Switch/3
  Switch/1 -> Gear axes-cg transformation/1(FMt model)
  ua/1 -> gear position/1
  gear position/1 -> Switch/2
  terr elev/1 -> Landing Gear model/3(terrain elevation)

== system Citation_FlightGear/Cessna Citation 500/Citation model DASMAT/AIRCRAFT MODEL/OBSERVATIONS ==
  note: Modified by Alex : Flight-Path Subsystem from Ac_mod instead of Ac_modpc
  x : Inport
  xdot : Inport  Port=2
  yuvw : Inport  Port=3
  FMtot : Inport  Port=4
  FMa : Inport  Port=5
  Fgr : Inport  Port=6
  massinit : Inport  Port=7
  yatm : Inport  Port=8
  Acceleration : Subsystem
  Energy : Subsystem
  Flight-Path : Subsystem
  yacc : Outport
  yfp : Outport  Port=2
  ys : Outport  Port=3
  wires:
  yuvw/1 -> Flight-Path/3(yuvw)
  Flight-Path/1(yfp) -> yfp/1
  Energy/1(ys) -> ys/1
  Acceleration/1(yacc) -> yacc/1
  FMa/1 -> Acceleration/4(FMa)
  Fgr/1 -> Acceleration/5(Fgr)
  yatm/1 -> Energy/3(yatm)
  FMtot/1 -> Acceleration/3(FMtot)
  Acceleration/2(acc earth) -> Flight-Path/4(acc earth)
  x/1 -> Flight-Path/1(x), Energy/1(x), Acceleration/1(x)
  xdot/1 -> Flight-Path/2(xdot), Energy/2(xdot), Acceleration/2(xdot)
  massinit/1 -> Acceleration/6(massinit)

== system Citation_FlightGear/Cessna Citation 500/Citation model DASMAT/AIRCRAFT MODEL/WIND//TURBULENCE ==
  "x " : Inport
  Logarithmic Wind model : Subsystem
  Mux : Mux  Inputs=[12 3]
  Vwind transformation : S-Function  FunctionName=ac_axes  Parameters=3  SFunctionDeploymentMode=off  EnableBusSupport=off
  wind : Outport
  wires:
  Mux/1 -> Vwind transformation/1
  Vwind transformation/1 -> wind/1
  "x "/1 -> Mux/1, Logarithmic Wind model/1(In1)
  Logarithmic Wind model/1(Out1) -> Mux/2
